simulink model "Plant1"  (R2016b)
settings: Solver=ode45  StartTime=0.0  StopTime=20  RelTol=1e-3  EnableMultiTasking=on
libraries: fuzblock x1
settings Model: Creator=Huu Toan  LastModifiedBy=Truc
settings DataIOCC: LimitDataPoints=on  SaveFormat=Array  SignalLoggingSaveFormat=ModelDataLogs
settings OptimizationCC: InitFltsAndDblsToZero=on  LifeSpan=inf
settings DebuggingCC: SaveWithParameterizedLinksMsg=none  UnderspecifiedInitializationDetection=Classic  MergeDetectMultiDrivingBlocksExec=none  SignalResolutionControl=TryResolveAllWithWarning  SolverPrmCheckMsg=warning  MultiTaskDSMMsg=warning  MultiTaskCondExecSysMsg=none  SFUnexpectedBacktrackingDiag=warning  SFNoUnconditionalDefaultTransitionDiag=warning  SFExecutionAtInitializationDiag=none
settings HardwareCC: ProdBitPerPointer=32  ProdBitPerSizeT=32  ProdBitPerPtrDiffT=32  ProdLargestAtomicFloat=None  ProdIntDivRoundTo=Undefined  ProdEndianess=Unspecified  ProdWordSize=32  ProdHWDeviceType=32-bit Generic
settings ModelReferenceCC: PropagateSignalLabelsOutOfModel=off
settings GRTTargetCC: TargetFcnLib=ansi_tfl_tmw.mat  TargetLangStandard=C89/C90 (ANSI)  CombineOutputUpdateFcns=off  GRTInterface=on
settings ConfigComp: CovMetricSettings=dw  CovHtmlReporting=on  CovSaveCumulativeToWorkspaceVar=on  CovSaveSingleToWorkspaceVar=on  CovExternalEMLEnable=off

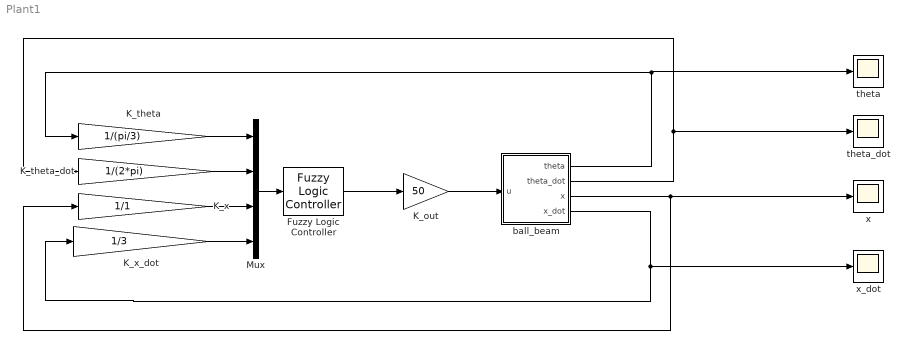
== system Plant1 ==
  Fuzzy Logic Controller : fuzblock/Fuzzy Logic  Controller  fis='ballbeam.fis'
  K_out : Gain  Gain=50
  K_theta : Gain  Gain=1/(pi/3)
  K_theta_dot : Gain  Gain=1/(2*pi)
  K_x : Gain  Gain=1/1
  K_x_dot : Gain  Gain=1/3
  Mux : Mux
  ball_beam : Subsystem  mask{m=0.3, J=0.00002, R=0.03, JB=0.2, g=9.81, init_cond=[pi/4 0 0.4 0]}
      mask prompts: m "Ball mass"; J "Ball moment"; R "Ball radius"; JB "Beam moment"; g "Gravity"; init_cond "Initial condition"
  theta : Scope
  theta_dot : Scope
  x : Scope
  x_dot : Scope
  wires:
  Mux/1 -> Fuzzy Logic Controller/1
  ball_beam/1(theta) -> K_theta/1, theta/1
  ball_beam/2(theta_dot) -> K_theta_dot/1, theta_dot/1
  ball_beam/3(x) -> K_x/1, x/1
  ball_beam/4(x_dot) -> K_x_dot/1, x_dot/1
  K_theta/1 -> Mux/1
  K_x/1 -> Mux/3
  K_x_dot/1 -> Mux/4
  K_theta_dot/1 -> Mux/2
  Fuzzy Logic Controller/1 -> K_out/1
  K_out/1 -> ball_beam/1(u)

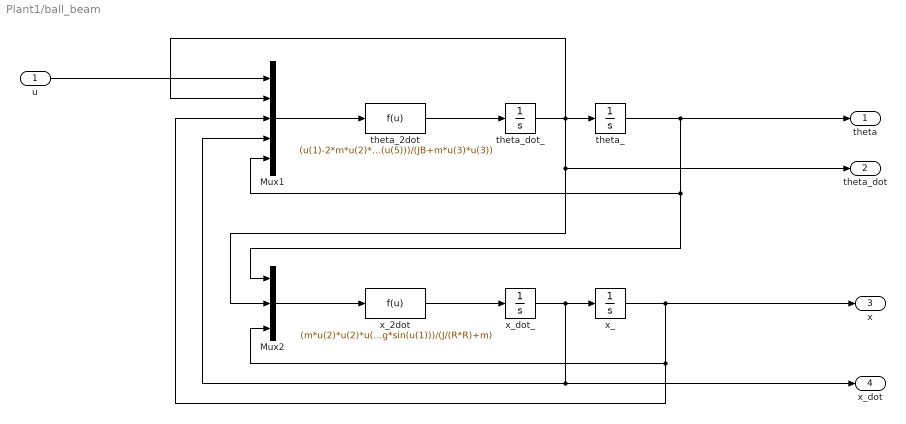
== system Plant1/ball_beam ==
  u : Inport
  Mux1 : Mux  Inputs=5
  Mux2 : Mux  Inputs=3
  theta_ : Integrator  InitialCondition=init_cond(1)
  theta_2dot : Fcn  Expr=(u(1)-2*m*u(2)*u(3)*u(4)-m*g*u(3)*cos(u(5)))/(JB+m*u(3)*u(3))
  theta_dot_ : Integrator  InitialCondition=init_cond(2)
  x_ : Integrator  InitialCondition=init_cond(3)
  x_2dot : Fcn  Expr=(m*u(2)*u(2)*u(3)-m*g*sin(u(1)))/(J/(R*R)+m)
  x_dot_ : Integrator  InitialCondition=init_cond(4)
  theta : Outport
  theta_dot : Outport  Port=2
  x : Outport  Port=3
  x_dot : Outport  Port=4
  wires:
  theta_2dot/1 -> theta_dot_/1
  u/1 -> Mux1/1
  Mux1/1 -> theta_2dot/1
  theta_dot_/1 -> theta_/1, Mux1/2, theta_dot/1, Mux2/2
  theta_/1 -> theta/1, Mux2/1, Mux1/5
  x_2dot/1 -> x_dot_/1
  x_dot_/1 -> x_/1, x_dot/1, Mux1/4
  Mux2/1 -> x_2dot/1
  x_/1 -> x/1, Mux1/3, Mux2/3
